simulink model "correct_sm_rectangle (1)"  (R2022b)
settings: Solver=VariableStepAuto  StartTime=0.0  StopTime=120  RelTol=1e-3
values from neighbouring files (symbols this model uses):
  Fxg = 0.005    [constants (3).m]
  Fyg = 0.005    [constants (3).m]
  g = 9.81    [constants (3).m]
  Ixx = 2.3951 * 10^-5    (= 2.3951e-05)    [constants (3).m]
  Iyy = 2.3951 * 10^-5    (= 2.3951e-05)    [constants (3).m]
  Izz = 3.2347 * 10^-5    (= 3.2347e-05)    [constants (3).m]
  kf = 0.005022    [constants (3).m]
  km = 1.858*10^-5    (= 1.858e-05)    [constants (3).m]
  L = 32 * 10^-3    (= 0.032)    [constants (3).m]
  m = 0.034    [constants (3).m]
libraries: slpidlib x6, matrix_library x1, aerolibutil x1
settings Model: Creator=nayan  LastModifiedBy=Sreejeet Maity
settings ModelReferenceCC: EnableRefExpFcnMdlSchedulingChecks=on

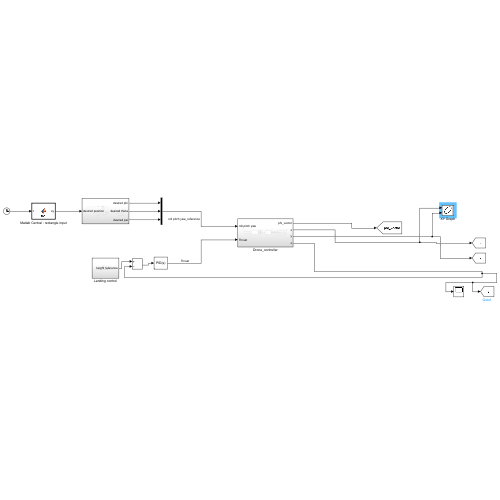
[thumbnail: Simulink's stored preview of the top-level diagram]
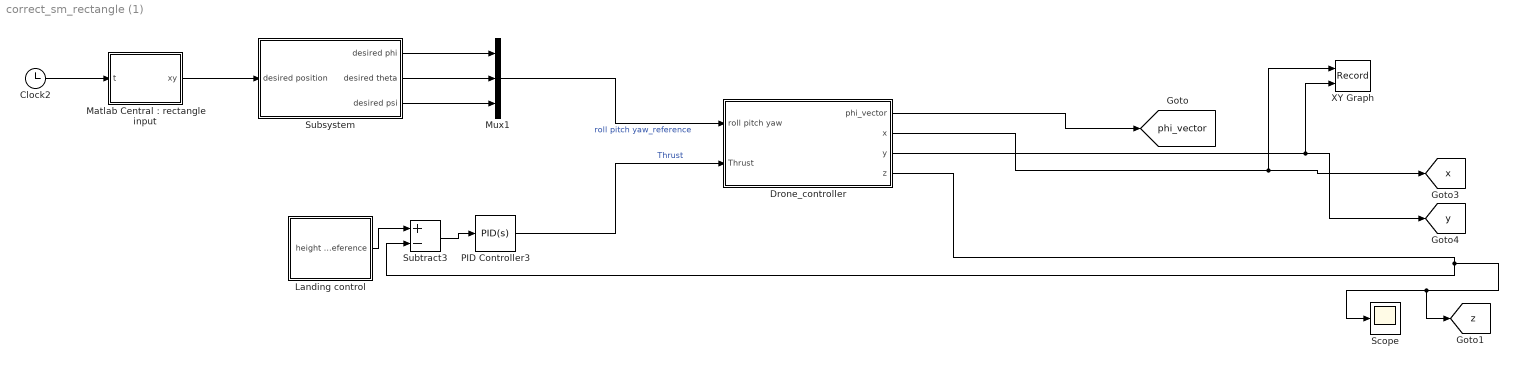
== system correct_sm_rectangle (1) ==
  Clock2 : Clock
  Drone_controller : Subsystem
  Landing control : Subsystem
  "Matlab Central : rectangle input" : MATLAB Function  TreatAsAtomicUnit=on
  Mux1 : Mux  Inputs=3
  PID Controller3 : slpidlib/PID Controller  Controller=PID  Form=Parallel  TimeDomain=Continuous-time  UseExternalTs=off  SampleTime=-1  IntegratorMethod=Forward Euler  FilterMethod=Forward Euler  ControllerParametersSource=internal  P=281.23  I=47.32  UseKiTs=off  D=18.56  N=1500  UseFilter=on  TunerSelectOption=Transfer Function Based (PID Tuner App)  InitialConditionSource=internal  InitialConditionForIntegrator=0  InitialConditionForFilter=0  DifferentiatorICPrevScaledInput=0  ExternalReset=none  TrackingMode=off  Kt=1  LimitOutput=off  SatLimitsSource=internal  UpperSaturationLimit=inf  LowerSaturationLimit=-inf  LinearizeAsGain=on  AntiWindupMode=none  Kb=1  LimitIntegrator=off  UpperIntegratorSaturationLimit=inf  LowerIntegratorSaturationLimit=-inf  POutMin=[]  POutMax=[]  IOutMin=[]  IOutMax=[]  DOutMin=[]  DOutMax=[]  NOutMin=[]  NOutMax=[]  SumOutMin=[]  SumOutMax=[]  SaturationOutMin=[]  SaturationOutMax=[]  PParamMin=[]  PParamMax=[]  IParamMin=[]  IParamMax=[]  DParamMin=[]  DParamMax=[]  NParamMin=[]  NParamMax=[]  KbParamMin=[]  KbParamMax=[]  KtParamMin=[]  KtParamMax=[]  KbOutMin=[]  KbOutMax=[]  KtOutMin=[]  KtOutMax=[]  IntegratorOutMin=[]  IntegratorOutMax=[]  FilterOutMin=[]  FilterOutMax=[]  SumI1OutMin=[]  SumI1OutMax=[]  SumI2OutMin=[]  SumI2OutMax=[]  SumI3OutMin=[]  SumI3OutMax=[]  SumI4OutMin=[]  SumI4OutMax=[]  SumDOutMin=[]  SumDOutMax=[]  DifferentiatorOutMin=[]  DifferentiatorOutMax=[]  FilterDiffOutCoefMin=[]  FilterDiffOutCoefMax=[]  ReciprocalOutMin=[]  ReciprocalOutMax=[]  SumDenOutMin=[]  SumDenOutMax=[]  SumNumOutMin=[]  SumNumOutMax=[]  DivideOutMin=[]  DivideOutMax=[]  UdiffTsProdOutMin=[]  UdiffTsProdOutMax=[]  NTsProdOutMin=[]  NTsProdOutMax=[]  UintegralTsProdOutMin=[]  UintegralTsProdOutMax=[]  UngainTsProdOutMin=[]  UngainTsProdOutMax=[]  ClampingZeroOutDataTypeStr=Inherit: Inherit via back propagation  ClampingZeroOutMin=[]  ClampingZeroOutMax=[]  FilterDenConstantOutDataTypeStr=Inherit: Inherit via back propagation  FilterDenConstantOutMin=[]  FilterDenConstantOutMax=[]  PCopyOutDataTypeStr=Inherit: Inherit via back propagation  PCopyOutMin=[]  PCopyOutMax=[]  NCopyOutDataTypeStr=Inherit: Inherit via back propagation  NCopyOutMin=[]  NCopyOutMax=[]  IntegratorContinuousStateAttributes=''  IntegratorStateMustResolveToSignalObject=off  IntegratorRTWStateStorageClass=Auto  FilterContinuousStateAttributes=''  FilterStateMustResolveToSignalObject=off  FilterRTWStateStorageClass=Auto  ParallelPVariant=InternalParameters  IdealPVariant=Disabled  IVariant=InternalParameters  DVariant=InternalParameters  IntegratorVariant=Continuous  SatVariant=Disabled  AWVariant=Passthrough  PCopyVariant=Disabled  TRVariant=Disabled  FdbkBlocksVariant=Forward  IdealPFdbkVariant=Disabled  SatFdbkVariant=Disabled  DerivativeFilterVariant=ContFilter  NVariant=InternalParameters  NCopyVariant=Disabled  FilterICVariant=InternalICsFilter  IntegratorICVariant=InternalICs  ExternalResetVariant=Disabled  TRSumVariant=Passthrough  SumFdbkVariant=Disabled  SumVariant=Sum_PID  TsampFilterVariant=InternalTs  TsampNgainVariant=Passthrough  TsampIntegralVariant=Passthrough  ExternalSaturationOutDataTypeStr=Inherit: Same as second input
  Scope : Scope
  Subsystem : Subsystem
  Subtract3 : Sum  Inputs=+-
  XY Graph : Record  FileSettingsInternal="{\"entries\":[{\"content\":{\"excelSettings\":{\"content\":{},\"type\":\"Streamout.ExcelSettings\"}},\"type\":\"Streamout.FileSettingStorage\",\"uuid\":\"9b419055-ec78-444e-b152-11d47a6ee07f\"}],\"packageUris\":[\"http://schema.mathworks.com/mf0/streamout_blocks/R2020a\"],\"version\":\"1.0\"}"  Layout=[1 1]  SignalsInternal="{\"entries\":[{\"content\":{\"signals\":[{\"content\":{\"blockPath\":[\"correct_sm_rectangle/XY Graph\"],\"channel\":[],\"dimensions\":[1],\"domain\":\"correct_sm_rectangle/XY Graph\",\"lineColor\":\"#a2142f\",\"plots\":[1],\"port\":1,\"sid\":[\"\"],\"signalID\":13322,\"signalName\":\"Drone_controller:2\"},\"type\":\"RecordBlkView.Signal\",\"uuid\":\"374e295a-d877-4438-a5ea-49d63ddf285e\"},{\"content\":{\"blockPath\":[\"correct_sm_rectangle/XY Graph\"],\"channel\":[],\"dimensions\":[1],\"domain\":\"correct_sm_rectangle/XY Graph\",\"lineColor\":\"#139fff\",\"plots\":[1],\"port\":2,\"sid\":[\"\"],\"signalID\":13326,\"signalName\":\"Drone_controller:3\"},\"type\":\"RecordBlkView.Signal\",\"uuid\":\"6c566137-3d76-4527-be06-b3cd4efedb4d\"}]},\"type\":\"RecordBlkView.InputSignals\",\"uuid\":\"8dcb939d-65f9-4e87-85f6-82af4bdaac8f\"}],\"packageUris\":[\"http://schema.mathworks.com/mf0/streamout_blocks/R2020a\"],\"version\":\"1.0\"}"  VisualizationBindings="{\"xyplotplugin\":{\"info\":[{\"series\":[{\"bindingParametersList\":[{\"parameter\":\"X-Axis\",\"signalID\":13322,\"signalName\":\"Drone_controller:2\"},{\"parameter\":\"Y-Axis\",\"signalID\":13326,\"signalName\":\"Drone_controller:3\"}],\"seriesID\":23091}],\"subplotID\":1}]}}"  CompatibilityTag=XY
  tag scope: phi_vector=global, x=global, y=global, z=global
  wires:
  Subsystem/1(desired phi) -> Mux1/1
  Subtract3/1 -> PID Controller3/1
  "Matlab Central : rectangle input"/1(xy) -> Subsystem/1(desired position)
  Subsystem/3(desired psi) -> Mux1/3
  Subsystem/2(desired theta) -> Mux1/2
  Clock2/1 -> "Matlab Central : rectangle input"/1(t)
  Landing control/1(height reference) -> Subtract3/1
  Drone_controller/2(x) -> XY Graph/1, [x]
  Drone_controller/4(z) -> [z], Scope/1, Subtract3/2
  Drone_controller/3(y) -> XY Graph/2, [y]
  Mux1/1 -> Drone_controller/1(roll pitch yaw)  "roll pitch yaw_reference"
  PID Controller3/1 -> Drone_controller/2(Thrust)  "Thrust"
  Drone_controller/1(phi_vector) -> [phi_vector]

== system correct_sm_rectangle (1)/Drone_controller ==
  roll pitch yaw : Inport
  Thrust : Inport  Port=2
  Attitude Controller : Subsystem
  Drone : Subsystem
  Mux : Mux
  phi_vector : Outport
  x : Outport  Port=2
  y : Outport  Port=3
  z : Outport  Port=4
  wires:
  Attitude Controller/3(w3_sqaure) -> Mux/3
  Mux/1 -> Drone/1(squares of omega)  "squares of motor rpm"
  Attitude Controller/1(w1_square) -> Mux/1
  roll pitch yaw/1 -> Attitude Controller/1(reference)
  Attitude Controller/4(w4_square) -> Mux/4
  Attitude Controller/2(w2_square) -> Mux/2
  Thrust/1 -> Attitude Controller/2(Thrust)
  Drone/4(z) -> z/1
  Drone/3(y) -> y/1
  Drone/2(x) -> x/1
  Drone/1(phi_vector) -> phi_vector/1

== system correct_sm_rectangle (1)/Landing control ==
  Clock : Clock
  Constant : Constant
  "Landing Time : 90 seconds" : Switch  Threshold=90  SaturateOnIntegerOverflow=off  InputSameDT=off
  Zero : Constant  Value=0  OutDataTypeStr=Inherit: Inherit via back propagation
  height reference : Outport
  wires:
  Constant/1 -> "Landing Time : 90 seconds"/3
  Zero/1 -> "Landing Time : 90 seconds"/1
  "Landing Time : 90 seconds"/1 -> height reference/1  "height reference"
  Clock/1 -> "Landing Time : 90 seconds"/2

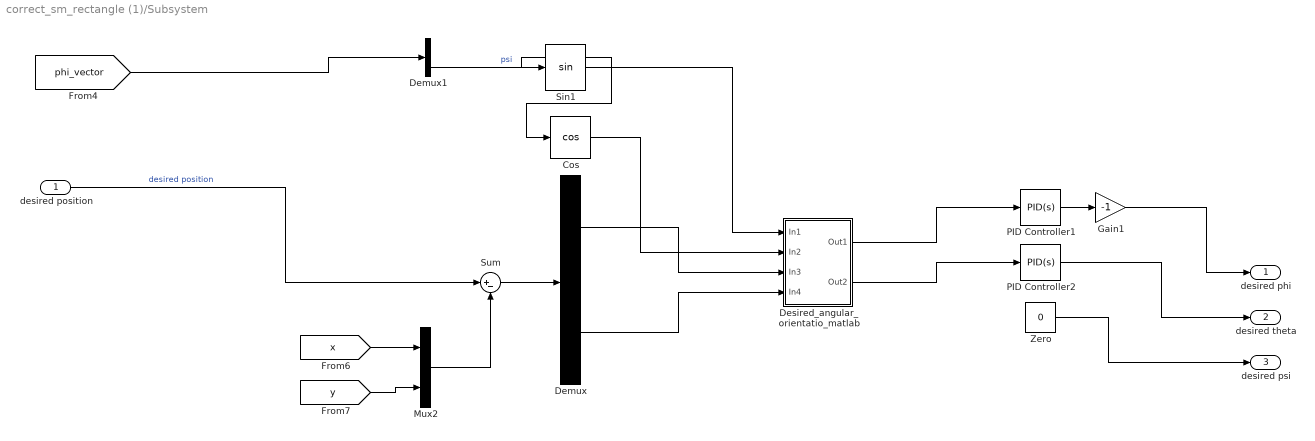
== system correct_sm_rectangle (1)/Subsystem ==
  desired position : Inport
  Cos : Trigonometry  Operator=cos
  Demux : Demux  Outputs=2
  Demux1 : Demux  Outputs=3
  Desired_angular_orientatio_matlab : Subsystem
  Gain1 : Gain  Gain=-1
  Mux2 : Mux  Inputs=2
  PID Controller1 : slpidlib/PID Controller  Controller=PID  Form=Parallel  TimeDomain=Continuous-time  UseExternalTs=off  SampleTime=-1  IntegratorMethod=Forward Euler  FilterMethod=Forward Euler  ControllerParametersSource=internal  P=0.043  I=0.0078  UseKiTs=off  D=0.07  N=10000  UseFilter=on  TunerSelectOption=Transfer Function Based (PID Tuner App)  InitialConditionSource=internal  InitialConditionForIntegrator=0  InitialConditionForFilter=0  DifferentiatorICPrevScaledInput=0  ExternalReset=none  TrackingMode=off  Kt=1  LimitOutput=off  SatLimitsSource=internal  UpperSaturationLimit=inf  LowerSaturationLimit=-inf  LinearizeAsGain=on  AntiWindupMode=none  Kb=1  LimitIntegrator=off  UpperIntegratorSaturationLimit=inf  LowerIntegratorSaturationLimit=-inf  POutMin=[]  POutMax=[]  IOutMin=[]  IOutMax=[]  DOutMin=[]  DOutMax=[]  NOutMin=[]  NOutMax=[]  SumOutMin=[]  SumOutMax=[]  SaturationOutMin=[]  SaturationOutMax=[]  PParamMin=[]  PParamMax=[]  IParamMin=[]  IParamMax=[]  DParamMin=[]  DParamMax=[]  NParamMin=[]  NParamMax=[]  KbParamMin=[]  KbParamMax=[]  KtParamMin=[]  KtParamMax=[]  KbOutMin=[]  KbOutMax=[]  KtOutMin=[]  KtOutMax=[]  IntegratorOutMin=[]  IntegratorOutMax=[]  FilterOutMin=[]  FilterOutMax=[]  SumI1OutMin=[]  SumI1OutMax=[]  SumI2OutMin=[]  SumI2OutMax=[]  SumI3OutMin=[]  SumI3OutMax=[]  SumI4OutMin=[]  SumI4OutMax=[]  SumDOutMin=[]  SumDOutMax=[]  DifferentiatorOutMin=[]  DifferentiatorOutMax=[]  FilterDiffOutCoefMin=[]  FilterDiffOutCoefMax=[]  ReciprocalOutMin=[]  ReciprocalOutMax=[]  SumDenOutMin=[]  SumDenOutMax=[]  SumNumOutMin=[]  SumNumOutMax=[]  DivideOutMin=[]  DivideOutMax=[]  UdiffTsProdOutMin=[]  UdiffTsProdOutMax=[]  NTsProdOutMin=[]  NTsProdOutMax=[]  UintegralTsProdOutMin=[]  UintegralTsProdOutMax=[]  UngainTsProdOutMin=[]  UngainTsProdOutMax=[]  ClampingZeroOutDataTypeStr=Inherit: Inherit via back propagation  ClampingZeroOutMin=[]  ClampingZeroOutMax=[]  FilterDenConstantOutDataTypeStr=Inherit: Inherit via back propagation  FilterDenConstantOutMin=[]  FilterDenConstantOutMax=[]  PCopyOutDataTypeStr=Inherit: Inherit via back propagation  PCopyOutMin=[]  PCopyOutMax=[]  NCopyOutDataTypeStr=Inherit: Inherit via back propagation  NCopyOutMin=[]  NCopyOutMax=[]  IntegratorContinuousStateAttributes=''  IntegratorStateMustResolveToSignalObject=off  IntegratorRTWStateStorageClass=Auto  FilterContinuousStateAttributes=''  FilterStateMustResolveToSignalObject=off  FilterRTWStateStorageClass=Auto  ParallelPVariant=InternalParameters  IdealPVariant=Disabled  IVariant=InternalParameters  DVariant=InternalParameters  IntegratorVariant=Continuous  SatVariant=Disabled  AWVariant=Passthrough  PCopyVariant=Disabled  TRVariant=Disabled  FdbkBlocksVariant=Forward  IdealPFdbkVariant=Disabled  SatFdbkVariant=Disabled  DerivativeFilterVariant=ContFilter  NVariant=InternalParameters  NCopyVariant=Disabled  FilterICVariant=InternalICsFilter  IntegratorICVariant=InternalICs  ExternalResetVariant=Disabled  TRSumVariant=Passthrough  SumFdbkVariant=Disabled  SumVariant=Sum_PID  TsampFilterVariant=InternalTs  TsampNgainVariant=Passthrough  TsampIntegralVariant=Passthrough  ExternalSaturationOutDataTypeStr=Inherit: Same as second input
  PID Controller2 : slpidlib/PID Controller  Controller=PID  Form=Parallel  TimeDomain=Continuous-time  UseExternalTs=off  SampleTime=-1  IntegratorMethod=Forward Euler  FilterMethod=Forward Euler  ControllerParametersSource=internal  P=0.067  I=0.0067  UseKiTs=off  D=0.06  N=10000  UseFilter=on  TunerSelectOption=Transfer Function Based (PID Tuner App)  InitialConditionSource=internal  InitialConditionForIntegrator=0  InitialConditionForFilter=0  DifferentiatorICPrevScaledInput=0  ExternalReset=none  TrackingMode=off  Kt=1  LimitOutput=off  SatLimitsSource=internal  UpperSaturationLimit=inf  LowerSaturationLimit=-inf  LinearizeAsGain=on  AntiWindupMode=none  Kb=1  LimitIntegrator=off  UpperIntegratorSaturationLimit=inf  LowerIntegratorSaturationLimit=-inf  POutMin=[]  POutMax=[]  IOutMin=[]  IOutMax=[]  DOutMin=[]  DOutMax=[]  NOutMin=[]  NOutMax=[]  SumOutMin=[]  SumOutMax=[]  SaturationOutMin=[]  SaturationOutMax=[]  PParamMin=[]  PParamMax=[]  IParamMin=[]  IParamMax=[]  DParamMin=[]  DParamMax=[]  NParamMin=[]  NParamMax=[]  KbParamMin=[]  KbParamMax=[]  KtParamMin=[]  KtParamMax=[]  KbOutMin=[]  KbOutMax=[]  KtOutMin=[]  KtOutMax=[]  IntegratorOutMin=[]  IntegratorOutMax=[]  FilterOutMin=[]  FilterOutMax=[]  SumI1OutMin=[]  SumI1OutMax=[]  SumI2OutMin=[]  SumI2OutMax=[]  SumI3OutMin=[]  SumI3OutMax=[]  SumI4OutMin=[]  SumI4OutMax=[]  SumDOutMin=[]  SumDOutMax=[]  DifferentiatorOutMin=[]  DifferentiatorOutMax=[]  FilterDiffOutCoefMin=[]  FilterDiffOutCoefMax=[]  ReciprocalOutMin=[]  ReciprocalOutMax=[]  SumDenOutMin=[]  SumDenOutMax=[]  SumNumOutMin=[]  SumNumOutMax=[]  DivideOutMin=[]  DivideOutMax=[]  UdiffTsProdOutMin=[]  UdiffTsProdOutMax=[]  NTsProdOutMin=[]  NTsProdOutMax=[]  UintegralTsProdOutMin=[]  UintegralTsProdOutMax=[]  UngainTsProdOutMin=[]  UngainTsProdOutMax=[]  ClampingZeroOutDataTypeStr=Inherit: Inherit via back propagation  ClampingZeroOutMin=[]  ClampingZeroOutMax=[]  FilterDenConstantOutDataTypeStr=Inherit: Inherit via back propagation  FilterDenConstantOutMin=[]  FilterDenConstantOutMax=[]  PCopyOutDataTypeStr=Inherit: Inherit via back propagation  PCopyOutMin=[]  PCopyOutMax=[]  NCopyOutDataTypeStr=Inherit: Inherit via back propagation  NCopyOutMin=[]  NCopyOutMax=[]  IntegratorContinuousStateAttributes=''  IntegratorStateMustResolveToSignalObject=off  IntegratorRTWStateStorageClass=Auto  FilterContinuousStateAttributes=''  FilterStateMustResolveToSignalObject=off  FilterRTWStateStorageClass=Auto  ParallelPVariant=InternalParameters  IdealPVariant=Disabled  IVariant=InternalParameters  DVariant=InternalParameters  IntegratorVariant=Continuous  SatVariant=Disabled  AWVariant=Passthrough  PCopyVariant=Disabled  TRVariant=Disabled  FdbkBlocksVariant=Forward  IdealPFdbkVariant=Disabled  SatFdbkVariant=Disabled  DerivativeFilterVariant=ContFilter  NVariant=InternalParameters  NCopyVariant=Disabled  FilterICVariant=InternalICsFilter  IntegratorICVariant=InternalICs  ExternalResetVariant=Disabled  TRSumVariant=Passthrough  SumFdbkVariant=Disabled  SumVariant=Sum_PID  TsampFilterVariant=InternalTs  TsampNgainVariant=Passthrough  TsampIntegralVariant=Passthrough  ExternalSaturationOutDataTypeStr=Inherit: Same as second input
  Sin1 : Trigonometry
  Sum : Sum  Inputs=|+-
  Zero : Constant  Value=0  OutDataTypeStr=Inherit: Inherit via back propagation
  desired phi : Outport
  desired theta : Outport  Port=2
  desired psi : Outport  Port=3
  wires:
  Sum/1 -> Demux/1
  PID Controller2/1 -> desired theta/1
  PID Controller1/1 -> Gain1/1
  Gain1/1 -> desired phi/1
  Demux1/3 -> Cos/1, Sin1/1  "psi"
  [x] -> Mux2/1
  Mux2/1 -> Sum/2
  [y] -> Mux2/2
  [phi_vector] -> Demux1/1
  desired position/1 -> Sum/1  "desired position"
  Zero/1 -> desired psi/1
  Sin1/1 -> Desired_angular_orientatio_matlab/1(In1)
  Cos/1 -> Desired_angular_orientatio_matlab/2(In2)
  Demux/1 -> Desired_angular_orientatio_matlab/3(In3)
  Demux/2 -> Desired_angular_orientatio_matlab/4(In4)
  Desired_angular_orientatio_matlab/1(Out1) -> PID Controller1/1
  Desired_angular_orientatio_matlab/2(Out2) -> PID Controller2/1

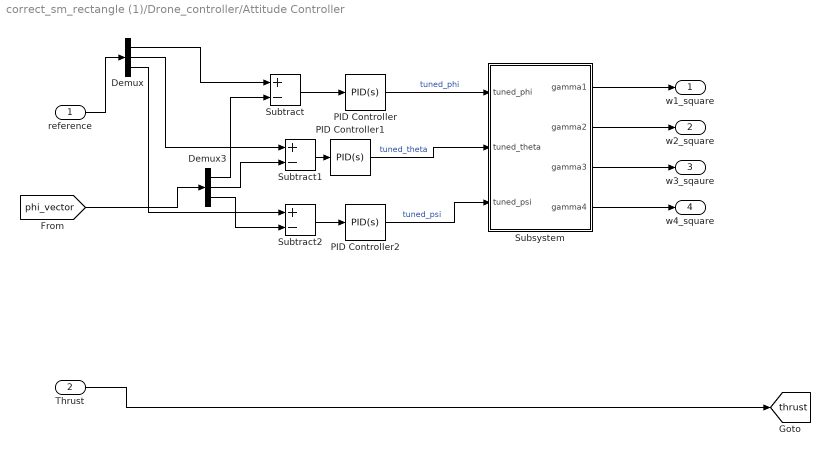
== system correct_sm_rectangle (1)/Drone_controller/Attitude Controller ==
  reference : Inport
  Thrust : Inport  Port=2
  Demux : Demux  Outputs=3
  Demux3 : Demux  Outputs=3
  PID Controller : slpidlib/PID Controller  Controller=PID  Form=Parallel  TimeDomain=Continuous-time  UseExternalTs=off  SampleTime=-1  IntegratorMethod=Forward Euler  FilterMethod=Forward Euler  ControllerParametersSource=internal  P=114.76  I=143  UseKiTs=off  D=40  N=10000  UseFilter=on  TunerSelectOption=Transfer Function Based (PID Tuner App)  InitialConditionSource=internal  InitialConditionForIntegrator=0  InitialConditionForFilter=0  DifferentiatorICPrevScaledInput=0  ExternalReset=none  TrackingMode=off  Kt=1  LimitOutput=off  SatLimitsSource=internal  UpperSaturationLimit=inf  LowerSaturationLimit=-inf  LinearizeAsGain=on  AntiWindupMode=none  Kb=1  LimitIntegrator=off  UpperIntegratorSaturationLimit=inf  LowerIntegratorSaturationLimit=-inf  POutMin=[]  POutMax=[]  IOutMin=[]  IOutMax=[]  DOutMin=[]  DOutMax=[]  NOutMin=[]  NOutMax=[]  SumOutMin=[]  SumOutMax=[]  SaturationOutMin=[]  SaturationOutMax=[]  PParamMin=[]  PParamMax=[]  IParamMin=[]  IParamMax=[]  DParamMin=[]  DParamMax=[]  NParamMin=[]  NParamMax=[]  KbParamMin=[]  KbParamMax=[]  KtParamMin=[]  KtParamMax=[]  KbOutMin=[]  KbOutMax=[]  KtOutMin=[]  KtOutMax=[]  IntegratorOutMin=[]  IntegratorOutMax=[]  FilterOutMin=[]  FilterOutMax=[]  SumI1OutMin=[]  SumI1OutMax=[]  SumI2OutMin=[]  SumI2OutMax=[]  SumI3OutMin=[]  SumI3OutMax=[]  SumI4OutMin=[]  SumI4OutMax=[]  SumDOutMin=[]  SumDOutMax=[]  DifferentiatorOutMin=[]  DifferentiatorOutMax=[]  FilterDiffOutCoefMin=[]  FilterDiffOutCoefMax=[]  ReciprocalOutMin=[]  ReciprocalOutMax=[]  SumDenOutMin=[]  SumDenOutMax=[]  SumNumOutMin=[]  SumNumOutMax=[]  DivideOutMin=[]  DivideOutMax=[]  UdiffTsProdOutMin=[]  UdiffTsProdOutMax=[]  NTsProdOutMin=[]  NTsProdOutMax=[]  UintegralTsProdOutMin=[]  UintegralTsProdOutMax=[]  UngainTsProdOutMin=[]  UngainTsProdOutMax=[]  ClampingZeroOutDataTypeStr=Inherit: Inherit via back propagation  ClampingZeroOutMin=[]  ClampingZeroOutMax=[]  FilterDenConstantOutDataTypeStr=Inherit: Inherit via back propagation  FilterDenConstantOutMin=[]  FilterDenConstantOutMax=[]  PCopyOutDataTypeStr=Inherit: Inherit via back propagation  PCopyOutMin=[]  PCopyOutMax=[]  NCopyOutDataTypeStr=Inherit: Inherit via back propagation  NCopyOutMin=[]  NCopyOutMax=[]  IntegratorContinuousStateAttributes=''  IntegratorStateMustResolveToSignalObject=off  IntegratorRTWStateStorageClass=Auto  FilterContinuousStateAttributes=''  FilterStateMustResolveToSignalObject=off  FilterRTWStateStorageClass=Auto  ParallelPVariant=InternalParameters  IdealPVariant=Disabled  IVariant=InternalParameters  DVariant=InternalParameters  IntegratorVariant=Continuous  SatVariant=Disabled  AWVariant=Passthrough  PCopyVariant=Disabled  TRVariant=Disabled  FdbkBlocksVariant=Forward  IdealPFdbkVariant=Disabled  SatFdbkVariant=Disabled  DerivativeFilterVariant=ContFilter  NVariant=InternalParameters  NCopyVariant=Disabled  FilterICVariant=InternalICsFilter  IntegratorICVariant=InternalICs  ExternalResetVariant=Disabled  TRSumVariant=Passthrough  SumFdbkVariant=Disabled  SumVariant=Sum_PID  TsampFilterVariant=InternalTs  TsampNgainVariant=Passthrough  TsampIntegralVariant=Passthrough  ExternalSaturationOutDataTypeStr=Inherit: Same as second input
  PID Controller1 : slpidlib/PID Controller  Controller=PID  Form=Parallel  TimeDomain=Continuous-time  UseExternalTs=off  SampleTime=-1  IntegratorMethod=Forward Euler  FilterMethod=Forward Euler  ControllerParametersSource=internal  P=114.76  I=143  UseKiTs=off  D=40  N=10000  UseFilter=on  TunerSelectOption=Transfer Function Based (PID Tuner App)  InitialConditionSource=internal  InitialConditionForIntegrator=0  InitialConditionForFilter=0  DifferentiatorICPrevScaledInput=0  ExternalReset=none  TrackingMode=off  Kt=1  LimitOutput=off  SatLimitsSource=internal  UpperSaturationLimit=inf  LowerSaturationLimit=-inf  LinearizeAsGain=on  AntiWindupMode=none  Kb=1  LimitIntegrator=off  UpperIntegratorSaturationLimit=inf  LowerIntegratorSaturationLimit=-inf  POutMin=[]  POutMax=[]  IOutMin=[]  IOutMax=[]  DOutMin=[]  DOutMax=[]  NOutMin=[]  NOutMax=[]  SumOutMin=[]  SumOutMax=[]  SaturationOutMin=[]  SaturationOutMax=[]  PParamMin=[]  PParamMax=[]  IParamMin=[]  IParamMax=[]  DParamMin=[]  DParamMax=[]  NParamMin=[]  NParamMax=[]  KbParamMin=[]  KbParamMax=[]  KtParamMin=[]  KtParamMax=[]  KbOutMin=[]  KbOutMax=[]  KtOutMin=[]  KtOutMax=[]  IntegratorOutMin=[]  IntegratorOutMax=[]  FilterOutMin=[]  FilterOutMax=[]  SumI1OutMin=[]  SumI1OutMax=[]  SumI2OutMin=[]  SumI2OutMax=[]  SumI3OutMin=[]  SumI3OutMax=[]  SumI4OutMin=[]  SumI4OutMax=[]  SumDOutMin=[]  SumDOutMax=[]  DifferentiatorOutMin=[]  DifferentiatorOutMax=[]  FilterDiffOutCoefMin=[]  FilterDiffOutCoefMax=[]  ReciprocalOutMin=[]  ReciprocalOutMax=[]  SumDenOutMin=[]  SumDenOutMax=[]  SumNumOutMin=[]  SumNumOutMax=[]  DivideOutMin=[]  DivideOutMax=[]  UdiffTsProdOutMin=[]  UdiffTsProdOutMax=[]  NTsProdOutMin=[]  NTsProdOutMax=[]  UintegralTsProdOutMin=[]  UintegralTsProdOutMax=[]  UngainTsProdOutMin=[]  UngainTsProdOutMax=[]  ClampingZeroOutDataTypeStr=Inherit: Inherit via back propagation  ClampingZeroOutMin=[]  ClampingZeroOutMax=[]  FilterDenConstantOutDataTypeStr=Inherit: Inherit via back propagation  FilterDenConstantOutMin=[]  FilterDenConstantOutMax=[]  PCopyOutDataTypeStr=Inherit: Inherit via back propagation  PCopyOutMin=[]  PCopyOutMax=[]  NCopyOutDataTypeStr=Inherit: Inherit via back propagation  NCopyOutMin=[]  NCopyOutMax=[]  IntegratorContinuousStateAttributes=''  IntegratorStateMustResolveToSignalObject=off  IntegratorRTWStateStorageClass=Auto  FilterContinuousStateAttributes=''  FilterStateMustResolveToSignalObject=off  FilterRTWStateStorageClass=Auto  ParallelPVariant=InternalParameters  IdealPVariant=Disabled  IVariant=InternalParameters  DVariant=InternalParameters  IntegratorVariant=Continuous  SatVariant=Disabled  AWVariant=Passthrough  PCopyVariant=Disabled  TRVariant=Disabled  FdbkBlocksVariant=Forward  IdealPFdbkVariant=Disabled  SatFdbkVariant=Disabled  DerivativeFilterVariant=ContFilter  NVariant=InternalParameters  NCopyVariant=Disabled  FilterICVariant=InternalICsFilter  IntegratorICVariant=InternalICs  ExternalResetVariant=Disabled  TRSumVariant=Passthrough  SumFdbkVariant=Disabled  SumVariant=Sum_PID  TsampFilterVariant=InternalTs  TsampNgainVariant=Passthrough  TsampIntegralVariant=Passthrough  ExternalSaturationOutDataTypeStr=Inherit: Same as second input
  PID Controller2 : slpidlib/PID Controller  Controller=PID  Form=Parallel  TimeDomain=Continuous-time  UseExternalTs=off  SampleTime=-1  IntegratorMethod=Forward Euler  FilterMethod=Forward Euler  ControllerParametersSource=internal  P=114.76  I=143  UseKiTs=off  D=40  N=10000  UseFilter=on  TunerSelectOption=Transfer Function Based (PID Tuner App)  InitialConditionSource=internal  InitialConditionForIntegrator=0  InitialConditionForFilter=0  DifferentiatorICPrevScaledInput=0  ExternalReset=none  TrackingMode=off  Kt=1  LimitOutput=off  SatLimitsSource=internal  UpperSaturationLimit=inf  LowerSaturationLimit=-inf  LinearizeAsGain=on  AntiWindupMode=none  Kb=1  LimitIntegrator=off  UpperIntegratorSaturationLimit=inf  LowerIntegratorSaturationLimit=-inf  POutMin=[]  POutMax=[]  IOutMin=[]  IOutMax=[]  DOutMin=[]  DOutMax=[]  NOutMin=[]  NOutMax=[]  SumOutMin=[]  SumOutMax=[]  SaturationOutMin=[]  SaturationOutMax=[]  PParamMin=[]  PParamMax=[]  IParamMin=[]  IParamMax=[]  DParamMin=[]  DParamMax=[]  NParamMin=[]  NParamMax=[]  KbParamMin=[]  KbParamMax=[]  KtParamMin=[]  KtParamMax=[]  KbOutMin=[]  KbOutMax=[]  KtOutMin=[]  KtOutMax=[]  IntegratorOutMin=[]  IntegratorOutMax=[]  FilterOutMin=[]  FilterOutMax=[]  SumI1OutMin=[]  SumI1OutMax=[]  SumI2OutMin=[]  SumI2OutMax=[]  SumI3OutMin=[]  SumI3OutMax=[]  SumI4OutMin=[]  SumI4OutMax=[]  SumDOutMin=[]  SumDOutMax=[]  DifferentiatorOutMin=[]  DifferentiatorOutMax=[]  FilterDiffOutCoefMin=[]  FilterDiffOutCoefMax=[]  ReciprocalOutMin=[]  ReciprocalOutMax=[]  SumDenOutMin=[]  SumDenOutMax=[]  SumNumOutMin=[]  SumNumOutMax=[]  DivideOutMin=[]  DivideOutMax=[]  UdiffTsProdOutMin=[]  UdiffTsProdOutMax=[]  NTsProdOutMin=[]  NTsProdOutMax=[]  UintegralTsProdOutMin=[]  UintegralTsProdOutMax=[]  UngainTsProdOutMin=[]  UngainTsProdOutMax=[]  ClampingZeroOutDataTypeStr=Inherit: Inherit via back propagation  ClampingZeroOutMin=[]  ClampingZeroOutMax=[]  FilterDenConstantOutDataTypeStr=Inherit: Inherit via back propagation  FilterDenConstantOutMin=[]  FilterDenConstantOutMax=[]  PCopyOutDataTypeStr=Inherit: Inherit via back propagation  PCopyOutMin=[]  PCopyOutMax=[]  NCopyOutDataTypeStr=Inherit: Inherit via back propagation  NCopyOutMin=[]  NCopyOutMax=[]  IntegratorContinuousStateAttributes=''  IntegratorStateMustResolveToSignalObject=off  IntegratorRTWStateStorageClass=Auto  FilterContinuousStateAttributes=''  FilterStateMustResolveToSignalObject=off  FilterRTWStateStorageClass=Auto  ParallelPVariant=InternalParameters  IdealPVariant=Disabled  IVariant=InternalParameters  DVariant=InternalParameters  IntegratorVariant=Continuous  SatVariant=Disabled  AWVariant=Passthrough  PCopyVariant=Disabled  TRVariant=Disabled  FdbkBlocksVariant=Forward  IdealPFdbkVariant=Disabled  SatFdbkVariant=Disabled  DerivativeFilterVariant=ContFilter  NVariant=InternalParameters  NCopyVariant=Disabled  FilterICVariant=InternalICsFilter  IntegratorICVariant=InternalICs  ExternalResetVariant=Disabled  TRSumVariant=Passthrough  SumFdbkVariant=Disabled  SumVariant=Sum_PID  TsampFilterVariant=InternalTs  TsampNgainVariant=Passthrough  TsampIntegralVariant=Passthrough  ExternalSaturationOutDataTypeStr=Inherit: Same as second input
  Subsystem : Subsystem
  Subtract : Sum  Inputs=+-
  Subtract1 : Sum  Inputs=+-
  Subtract2 : Sum  Inputs=+-
  w1_square : Outport
  w2_square : Outport  Port=2
  w3_sqaure : Outport  Port=3
  w4_square : Outport  Port=4
  tag scope: thrust=global
  wires:
  Subtract2/1 -> PID Controller2/1
  Demux3/2 -> Subtract1/2
  [phi_vector] -> Demux3/1
  Demux3/3 -> Subtract2/2
  Subtract1/1 -> PID Controller1/1
  Subtract/1 -> PID Controller/1
  Demux3/1 -> Subtract/2
  reference/1 -> Demux/1
  Demux/1 -> Subtract/1
  Demux/2 -> Subtract1/1
  Demux/3 -> Subtract2/1
  Thrust/1 -> [thrust]
  PID Controller/1 -> Subsystem/1(tuned_phi)  "tuned_phi"
  PID Controller1/1 -> Subsystem/2(tuned_theta)  "tuned_theta"
  PID Controller2/1 -> Subsystem/3(tuned_psi)  "tuned_psi"
  Subsystem/1(gamma1) -> w1_square/1
  Subsystem/2(gamma2) -> w2_square/1
  Subsystem/3(gamma3) -> w3_sqaure/1
  Subsystem/4(gamma4) -> w4_square/1

== system correct_sm_rectangle (1)/Drone_controller/Drone ==
  squares of omega : Inport
  Drone dynamics : Subsystem
  MMA : Subsystem
  phi_vector : Outport
  x : Outport  Port=2
  y : Outport  Port=3
  z : Outport  Port=4
  wires:
  Drone dynamics/4(z) -> z/1
  MMA/1(Thrust) -> Drone dynamics/1(Thrust)
  Drone dynamics/3(y) -> y/1
  MMA/2("[Tau_x;Tau_y;Tau_z]") -> Drone dynamics/2(tau_vector)
  Drone dynamics/1(phi_vector) -> phi_vector/1
  Drone dynamics/2(x) -> x/1
  squares of omega/1 -> MMA/1(omega_squares_vector)

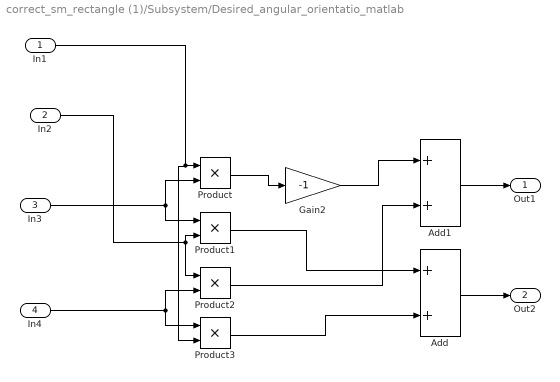
== system correct_sm_rectangle (1)/Subsystem/Desired_angular_orientatio_matlab ==
  In1 : Inport
  In2 : Inport  Port=2
  In3 : Inport  Port=3
  In4 : Inport  Port=4
  Add : Sum
  Add1 : Sum
  Gain2 : Gain  Gain=-1
  Product{,1..3} (4 alike) : Product
  Out1 : Outport
  Out2 : Outport  Port=2
  wires:
  Product3/1 -> Add/2
  Product/1 -> Gain2/1
  In4/1 -> Product2/2, Product3/1
  In3/1 -> Product1/1, Product/2
  In2/1 -> Product2/1, Product1/2
  Product2/1 -> Add1/2
  Add/1 -> Out2/1
  In1/1 -> Product3/2, Product/1
  Gain2/1 -> Add1/1
  Product1/1 -> Add/1
  Add1/1 -> Out1/1

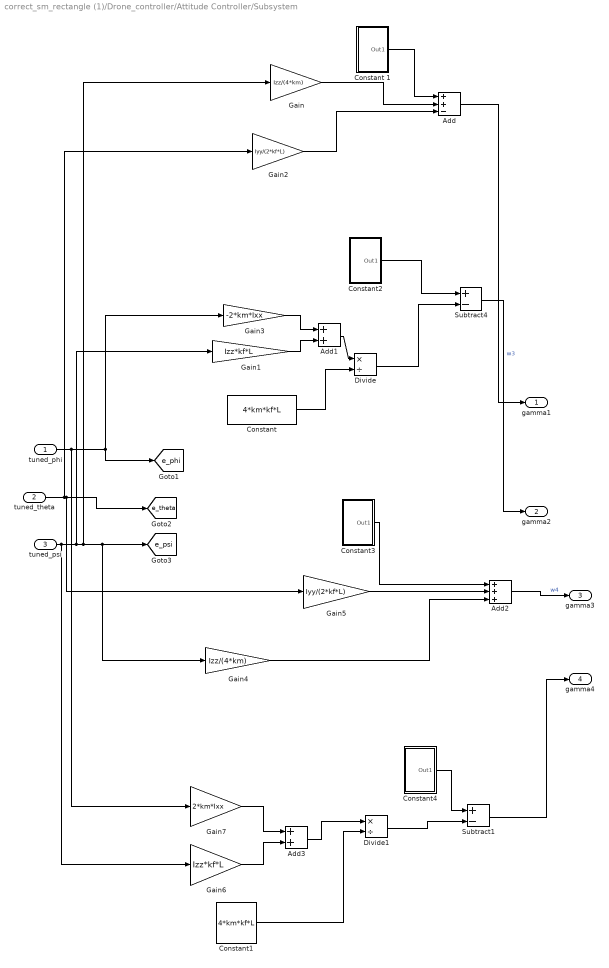
== system correct_sm_rectangle (1)/Drone_controller/Attitude Controller/Subsystem ==
  tuned_phi : Inport
  tuned_theta : Inport  Port=2
  tuned_psi : Inport  Port=3
  Add : Sum  Inputs=++-
  Add1 : Sum
  Add2 : Sum  Inputs=+++
  Add3 : Sum
  Constant : Constant  Value=4*km*kf*L
  Constant 1 : Subsystem
  Constant1 : Constant  Value=4*km*kf*L
  Constant2 : Subsystem
  Constant3 : Subsystem
  Constant4 : Subsystem
  Divide : Product  Inputs=*/
  Divide1 : Product  Inputs=*/
  Gain : Gain  Gain=Izz/(4*km)
  Gain1 : Gain  Gain=Izz*kf*L
  Gain2 : Gain  Gain=Iyy/(2*kf*L)
  Gain3 : Gain  Gain=-2*km*Ixx
  Gain4 : Gain  Gain=Izz/(4*km)
  Gain5 : Gain  Gain=Iyy/(2*kf*L)
  Gain6 : Gain  Gain=Izz*kf*L
  Gain7 : Gain  Gain=2*km*Ixx
  Subtract1 : Sum  Inputs=+-
  Subtract4 : Sum  Inputs=+-
  gamma1 : Outport
  gamma2 : Outport  Port=2
  gamma3 : Outport  Port=3
  gamma4 : Outport  Port=4
  tag scope: e_phi=global, e_psi=global, e_theta=global
  wires:
  Subtract1/1 -> gamma4/1
  Add/1 -> gamma1/1
  Gain2/1 -> Add/3
  Gain/1 -> Add/2
  Constant 1/1(Out1) -> Add/1
  Constant/1 -> Divide/2
  Add1/1 -> Divide/1
  Divide/1 -> Subtract4/2
  Gain3/1 -> Add1/1
  Subtract4/1 -> gamma2/1  "w3"
  Constant2/1(Out1) -> Subtract4/1
  Gain1/1 -> Add1/2
  Gain4/1 -> Add2/3
  tuned_theta/1 -> [e_theta], Gain5/1, Gain2/1
  Add2/1 -> gamma3/1  "w4"
  Gain5/1 -> Add2/2
  Constant3/1(Out1) -> Add2/1
  tuned_psi/1 -> [e_psi], Gain4/1, Gain/1, Gain1/1, Gain6/1
  Constant1/1 -> Divide1/2
  Constant4/1(Out1) -> Subtract1/1
  Gain6/1 -> Add3/2
  tuned_phi/1 -> Gain3/1, [e_phi], Gain7/1
  Divide1/1 -> Subtract1/2
  Gain7/1 -> Add3/1
  Add3/1 -> Divide1/1

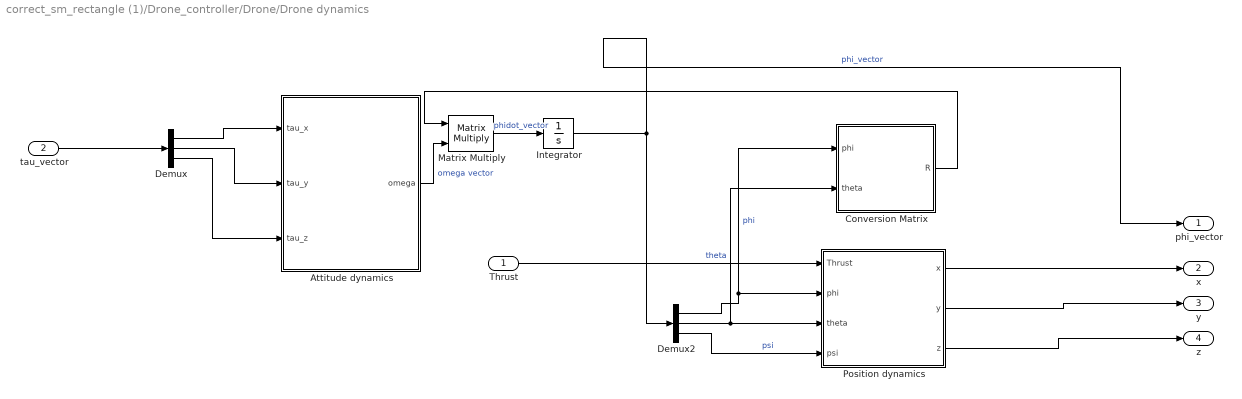
== system correct_sm_rectangle (1)/Drone_controller/Drone/Drone dynamics ==
  Thrust : Inport
  tau_vector : Inport  Port=2
  Attitude dynamics : Subsystem
  Conversion Matrix : MATLAB Function  TreatAsAtomicUnit=on
  Demux : Demux  Outputs=3
  Demux2 : Demux  Outputs=3
  Integrator : Integrator  WrapState=on
  Matrix Multiply : Product  Multiplication=Matrix(*)
  Position dynamics : Subsystem
  phi_vector : Outport
  x : Outport  Port=2
  y : Outport  Port=3
  z : Outport  Port=4
  wires:
  Attitude dynamics/1(omega) -> Matrix Multiply/2  "omega vector"
  Integrator/1 -> phi_vector/1, Demux2/1  "phi_vector"
  Demux2/2 -> Conversion Matrix/2(theta), Position dynamics/3(theta)  "theta"
  Matrix Multiply/1 -> Integrator/1  "phidot_vector"
  Demux2/1 -> Conversion Matrix/1(phi), Position dynamics/2(phi)  "phi"
  Demux2/3 -> Position dynamics/4(psi)  "psi"
  Thrust/1 -> Position dynamics/1(Thrust)
  Position dynamics/3(z) -> z/1
  Position dynamics/2(y) -> y/1
  Position dynamics/1(x) -> x/1
  Demux/1 -> Attitude dynamics/1(tau_x)
  Demux/2 -> Attitude dynamics/2(tau_y)
  Demux/3 -> Attitude dynamics/3(tau_z)
  tau_vector/1 -> Demux/1
  Conversion Matrix/1(R) -> Matrix Multiply/1

== system correct_sm_rectangle (1)/Drone_controller/Drone/MMA ==
  omega_squares_vector : Inport
  Constant : Constant  Value=[kf kf kf kf; 0 kf*L 0 -kf*L; -kf*L 0 kf*L 0; km -km km -km]
  Demux : Demux
  Matrix Multiply : Product  Multiplication=Matrix(*)
  Mux1 : Mux  Inputs=3
  Thrust : Outport
  "[Tau_x;Tau_y;Tau_z]" : Outport  Port=2
  wires:
  Demux/4 -> Mux1/3
  Demux/3 -> Mux1/2
  Demux/2 -> Mux1/1
  Mux1/1 -> "[Tau_x;Tau_y;Tau_z]"/1
  Demux/1 -> Thrust/1
  Matrix Multiply/1 -> Demux/1
  Constant/1 -> Matrix Multiply/1
  omega_squares_vector/1 -> Matrix Multiply/2

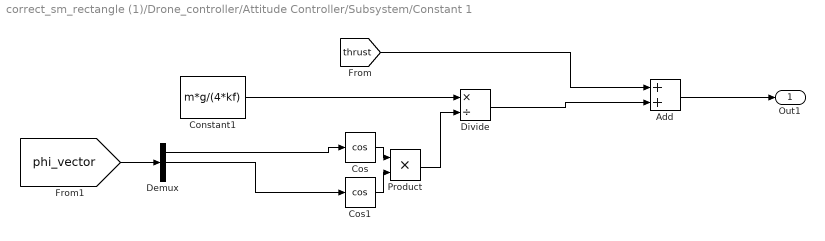
== system correct_sm_rectangle (1)/Drone_controller/Attitude Controller/Subsystem/Constant 1 ==
  Add : Sum
  Constant1 : Constant  Value=m*g/(4*kf)
  Cos : Trigonometry  Operator=cos
  Cos1 : Trigonometry  Operator=cos
  Demux : Demux  Outputs=3
  Divide : Product  Inputs=*/
  Product : Product
  Out1 : Outport
  wires:
  Add/1 -> Out1/1
  Cos1/1 -> Product/2
  Product/1 -> Divide/2
  Constant1/1 -> Divide/1
  Demux/2 -> Cos1/1
  Demux/1 -> Cos/1
  [phi_vector] -> Demux/1
  Divide/1 -> Add/2
  Cos/1 -> Product/1
  [thrust] -> Add/1

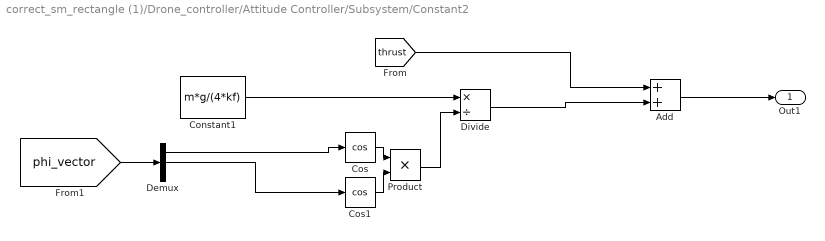
== system correct_sm_rectangle (1)/Drone_controller/Attitude Controller/Subsystem/Constant2 ==
  Add : Sum
  Constant1 : Constant  Value=m*g/(4*kf)
  Cos : Trigonometry  Operator=cos
  Cos1 : Trigonometry  Operator=cos
  Demux : Demux  Outputs=3
  Divide : Product  Inputs=*/
  Product : Product
  Out1 : Outport
  wires:
  Add/1 -> Out1/1
  Cos1/1 -> Product/2
  Product/1 -> Divide/2
  Constant1/1 -> Divide/1
  Demux/2 -> Cos1/1
  Demux/1 -> Cos/1
  [phi_vector] -> Demux/1
  Divide/1 -> Add/2
  Cos/1 -> Product/1
  [thrust] -> Add/1

== system correct_sm_rectangle (1)/Drone_controller/Attitude Controller/Subsystem/Constant3 ==
  Add : Sum
  Constant1 : Constant  Value=m*g/(4*kf)
  Cos : Trigonometry  Operator=cos
  Cos1 : Trigonometry  Operator=cos
  Demux : Demux  Outputs=3
  Divide : Product  Inputs=*/
  Product : Product
  Out1 : Outport
  wires:
  [thrust] -> Add/1
  Cos/1 -> Product/1
  Divide/1 -> Add/2
  [phi_vector] -> Demux/1
  Demux/1 -> Cos/1
  Demux/2 -> Cos1/1
  Constant1/1 -> Divide/1
  Product/1 -> Divide/2
  Cos1/1 -> Product/2
  Add/1 -> Out1/1

== system correct_sm_rectangle (1)/Drone_controller/Attitude Controller/Subsystem/Constant4 ==
  Add : Sum
  Constant1 : Constant  Value=m*g/(4*kf)
  Cos : Trigonometry  Operator=cos
  Cos1 : Trigonometry  Operator=cos
  Demux : Demux  Outputs=3
  Divide : Product  Inputs=*/
  Product : Product
  Out1 : Outport
  wires:
  Add/1 -> Out1/1
  Cos1/1 -> Product/2
  Product/1 -> Divide/2
  Constant1/1 -> Divide/1
  Demux/2 -> Cos1/1
  Demux/1 -> Cos/1
  [phi_vector] -> Demux/1
  Divide/1 -> Add/2
  Cos/1 -> Product/1
  [thrust] -> Add/1

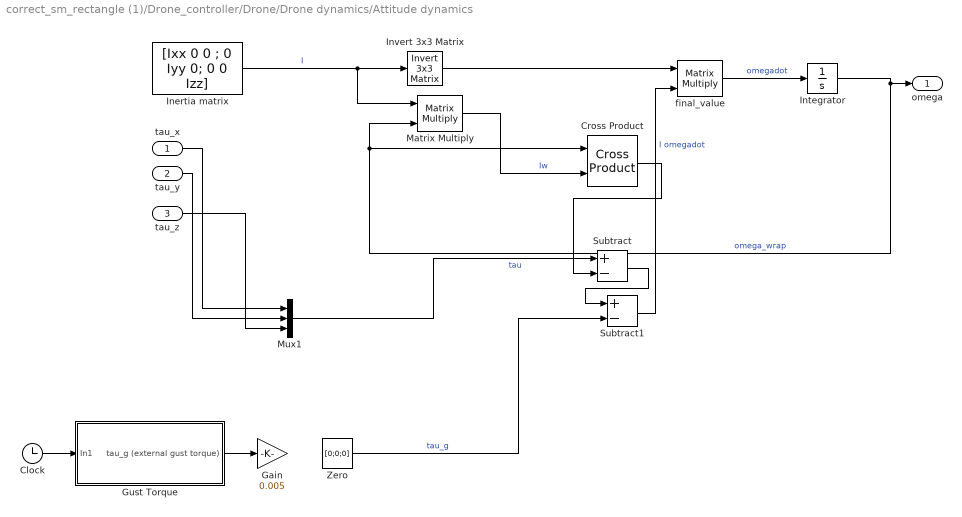
== system correct_sm_rectangle (1)/Drone_controller/Drone/Drone dynamics/Attitude dynamics ==
  tau_x : Inport
  tau_y : Inport  Port=2
  tau_z : Inport  Port=3
  Clock : Clock
  Cross Product : matrix_library/Cross Product
  Gain : Gain  Gain=0.005
  Gust Torque : Subsystem
  Inertia matrix : Constant  Value=[Ixx 0 0 ; 0 Iyy 0; 0 0 Izz]
  Integrator : Integrator  WrapState=on
  Invert 3x3 Matrix : aerolibutil/Invert  3x3 Matrix
  Matrix Multiply : Product  Multiplication=Matrix(*)
  Mux1 : Mux  Inputs=3
  Subtract : Sum  Inputs=+-
  Subtract1 : Sum  Inputs=+-
  Zero : Constant  Value=[0;0;0]  OutDataTypeStr=Inherit: Inherit via back propagation
  final_value : Product  Multiplication=Matrix(*)
  omega : Outport
  wires:
  Integrator/1 -> omega/1, Cross Product/1, Matrix Multiply/2  "omega_wrap"
  Matrix Multiply/1 -> Cross Product/2  "Iw"
  Inertia matrix/1 -> Invert 3x3 Matrix/1, Matrix Multiply/1  "I"
  Zero/1 -> Subtract1/2  "tau_g"
  Subtract/1 -> Subtract1/1
  Cross Product/1 -> Subtract/2
  Mux1/1 -> Subtract/1  "tau"
  tau_y/1 -> Mux1/2
  tau_z/1 -> Mux1/3
  tau_x/1 -> Mux1/1
  Subtract1/1 -> final_value/2  "I omegadot"
  Invert 3x3 Matrix/1 -> final_value/1
  final_value/1 -> Integrator/1  "omegadot"
  Clock/1 -> Gust Torque/1(In1)
  Gust Torque/1(tau_g (external gust torque)) -> Gain/1

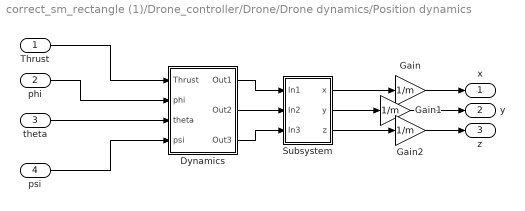
== system correct_sm_rectangle (1)/Drone_controller/Drone/Drone dynamics/Position dynamics ==
  Thrust : Inport
  phi : Inport  Port=2
  theta : Inport  Port=3
  psi : Inport  Port=4
  Dynamics : Subsystem
  Gain : Gain  Gain=1/m
  Gain1 : Gain  Gain=1/m
  Gain2 : Gain  Gain=1/m
  Subsystem : Subsystem
  x : Outport
  y : Outport  Port=2
  z : Outport  Port=3
  wires:
  Subsystem/1(x) -> Gain/1
  Subsystem/2(y) -> Gain1/1
  Subsystem/3(z) -> Gain2/1
  Thrust/1 -> Dynamics/1(Thrust)
  phi/1 -> Dynamics/2(phi)
  theta/1 -> Dynamics/3(theta)
  psi/1 -> Dynamics/4(psi)
  Dynamics/1(Out1) -> Subsystem/1(In1)
  Dynamics/2(Out2) -> Subsystem/2(In2)
  Dynamics/3(Out3) -> Subsystem/3(In3)
  Gain/1 -> x/1
  Gain1/1 -> y/1
  Gain2/1 -> z/1

== system correct_sm_rectangle (1)/Drone_controller/Drone/Drone dynamics/Attitude dynamics/Gust Torque ==
  In1 : Inport
  Cos : Trigonometry  Operator=cos
  Gain : Gain  Gain=2
  Mux2 : Mux  Inputs=3
  Sin : Trigonometry
  tau_g (external gust torque) : Outport
  wires:
  Cos/1 -> Mux2/1
  Sin/1 -> Gain/1, Mux2/2
  In1/1 -> Sin/1, Cos/1
  Gain/1 -> Mux2/3
  Mux2/1 -> tau_g (external gust torque)/1  "tau_g (external gust torque)"

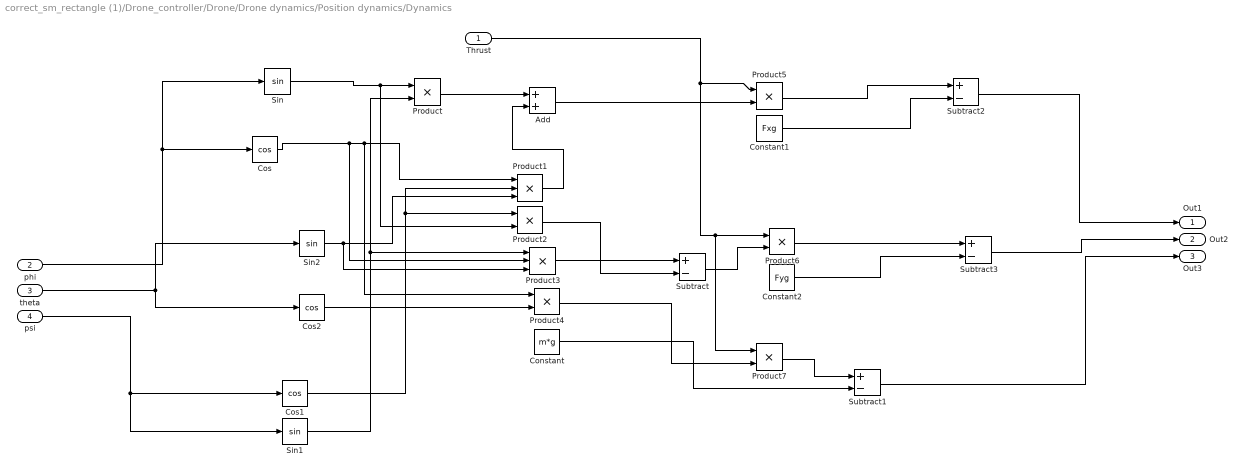
== system correct_sm_rectangle (1)/Drone_controller/Drone/Drone dynamics/Position dynamics/Dynamics ==
  Thrust : Inport
  phi : Inport  Port=2
  theta : Inport  Port=3
  psi : Inport  Port=4
  Add : Sum
  Constant : Constant  Value=m*g
  Constant1 : Constant  Value=Fxg
  Constant2 : Constant  Value=Fyg
  Cos : Trigonometry  Operator=cos
  Cos1 : Trigonometry  Operator=cos
  Cos2 : Trigonometry  Operator=cos
  Product{,2,4..7} (6 alike) : Product
  Product1 : Product  Inputs=3
  Product3 : Product  Inputs=3
  Sin : Trigonometry
  Sin1 : Trigonometry
  Sin2 : Trigonometry
  Subtract{,1..3} (4 alike) : Sum  Inputs=+-
  Out1 : Outport
  Out2 : Outport  Port=2
  Out3 : Outport  Port=3
  wires:
  phi/1 -> Sin/1, Cos/1
  Cos1/1 -> Product2/1, Product1/2
  Cos/1 -> Product3/2, Product4/1, Product1/1
  Product5/1 -> Subtract2/1
  Cos2/1 -> Product4/2
  psi/1 -> Sin1/1, Cos1/1
  Product6/1 -> Subtract3/1
  Thrust/1 -> Product7/1, Product6/1, Product5/1
  Product3/1 -> Subtract/1
  Product7/1 -> Subtract1/1
  Subtract/1 -> Product6/2
  Product4/1 -> Product7/2
  Subtract3/1 -> Out2/1
  Product1/1 -> Add/2
  Constant/1 -> Subtract1/2
  Sin2/1 -> Product3/3, Product1/3
  Add/1 -> Product5/2
  theta/1 -> Cos2/1, Sin2/1
  Subtract2/1 -> Out1/1
  Subtract1/1 -> Out3/1
  Constant2/1 -> Subtract3/2
  Product/1 -> Add/1
  Constant1/1 -> Subtract2/2
  Product2/1 -> Subtract/2
  Sin1/1 -> Product3/1, Product/2
  Sin/1 -> Product2/2, Product/1

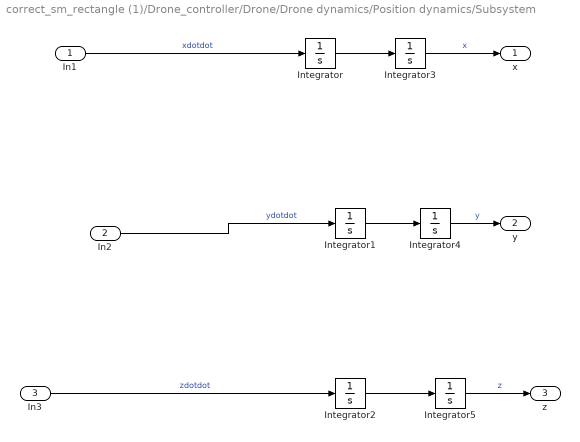
== system correct_sm_rectangle (1)/Drone_controller/Drone/Drone dynamics/Position dynamics/Subsystem ==
  In1 : Inport
  In2 : Inport  Port=2
  In3 : Inport  Port=3
  Integrator{,1..4} (5 alike) : Integrator
  Integrator5 : Integrator  LimitOutput=on  LowerSaturationLimit=0
  x : Outport
  y : Outport  Port=2
  z : Outport  Port=3
  wires:
  Integrator5/1 -> z/1  "z"
  In3/1 -> Integrator2/1  "zdotdot"
  Integrator2/1 -> Integrator5/1
  In2/1 -> Integrator1/1  "ydotdot"
  Integrator1/1 -> Integrator4/1
  In1/1 -> Integrator/1  "xdotdot"
  Integrator4/1 -> y/1  "y"
  Integrator/1 -> Integrator3/1
  Integrator3/1 -> x/1  "x"

== matlab function correct_sm_rectangle (1)/Matlab Central : rectangle input ==
  data: xy output; t input
function xy = fcn(t)

if t<=20
    xy=[1;1];
elseif (t>10) && (t<=30)
    xy=[2;1];
    elseif (t>30) && (t<=50)
    xy=[2;2];
    elseif (t>50) && (t<=70)
    xy=[1;2];
else xy=[1;1];
end

== matlab function correct_sm_rectangle (1)/Drone_controller/Drone/Drone dynamics/Conversion Matrix ==
  data: phi input; R output; theta input
function R = fcn(phi,theta)
R = [1 0 -sin(theta) ; 0 cos(phi) cos(theta)*sin(phi) ; 0 -sin(phi) cos(theta)*cos(phi)] ;
